simulink model "Subsystem"  (R2020b)
settings: Solver=VariableStepAuto  StartTime=0.0  StopTime=10.0  RelTol=1e-3
settings Model: Creator=shivanshu shukla  LastModifiedBy=shivanshu shukla
settings DataIOCC: SaveOutput=off  SaveTime=off

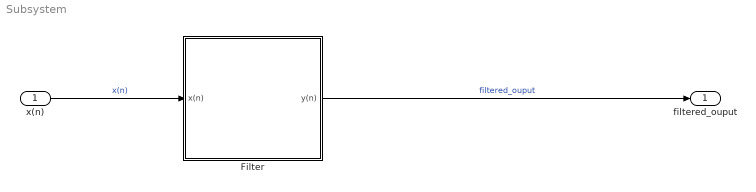
== system Subsystem ==
  x(n) : Inport  OutDataTypeStr=double  PortDimensions=1  SampleTime=[0,1]
  Filter : Subsystem
  filtered_ouput : Outport  OutDataTypeStr=double  PortDimensions=1  SampleTime=[0,1]
  wires:
  x(n)/1 -> Filter/1(x(n))  "x(n)"
  Filter/1(y(n)) -> filtered_ouput/1  "filtered_ouput"

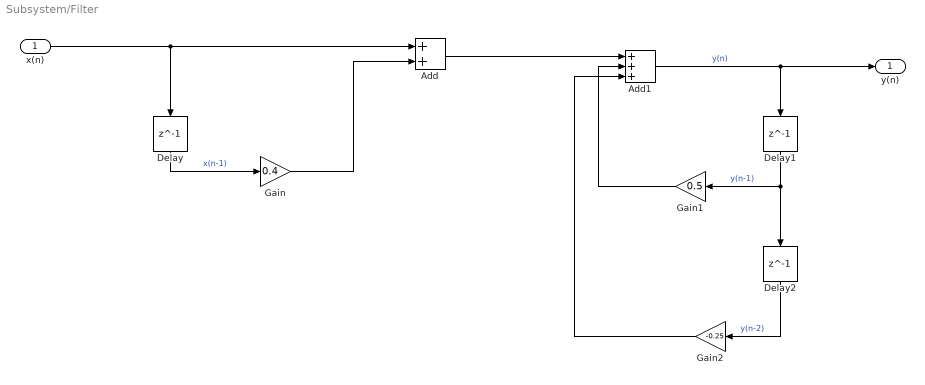
== system Subsystem/Filter ==
  x(n) : Inport
  Add : Sum
  Add1 : Sum  Inputs=+++
  Delay : Delay  DelayLength=1
  Delay1 : Delay  DelayLength=1
  Delay2 : Delay  DelayLength=1
  Gain : Gain  Gain=0.4
  Gain1 : Gain  Gain=0.5
  Gain2 : Gain  Gain=-0.25
  y(n) : Outport
  wires:
  Delay/1 -> Gain/1  "x(n-1)"
  x(n)/1 -> Delay/1, Add/1
  Delay1/1 -> Gain1/1, Delay2/1  "y(n-1)"
  Gain/1 -> Add/2
  Gain2/1 -> Add1/3
  Delay2/1 -> Gain2/1  "y(n-2)"
  Add/1 -> Add1/1
  Gain1/1 -> Add1/2
  Add1/1 -> Delay1/1, y(n)/1  "y(n)"
